simulink model "lineTwist"  (Simulink 8.5)
settings: Solver=ode15s  SolverMode=SingleTasking  StartTime=0.0  StopTime=0.1  MaxStep=0.0001  RelTol=1e-4  AbsTol=1e-6
libraries: powerlib x46
settings Model: Creator=Dr. Lotfifard  LastModifiedBy=PC
settings SolverCC: InitialStep=0.000001
settings DataIOCC: LimitDataPoints=off
settings OptimizationCC: BlockReduction=off  BooleanDataType=off
settings DebuggingCC: SaveWithParameterizedLinksMsg=none  SignalResolutionControl=TryResolveAllWithWarning  MultiTaskDSMMsg=warning  MultiTaskCondExecSysMsg=none  FcnCallInpInsideContextMsg=UseLocalSettings
settings HardwareCC: TargetUnknown=on

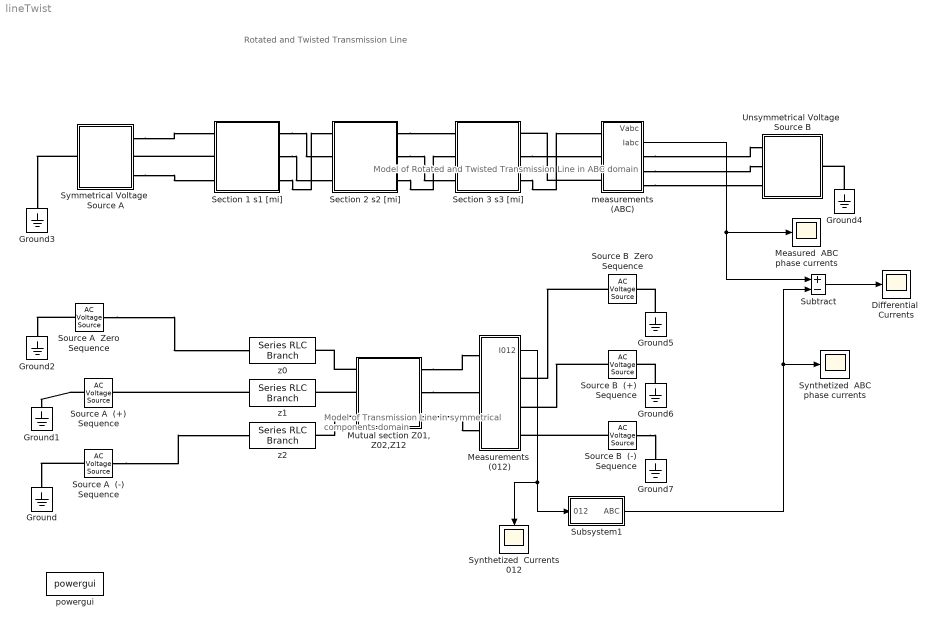
== system lineTwist ==
  note: Rotated and Twisted Transmission Line
  note: Model of Transmission Line
      |     in symmetrical components domain
  note: Model of Rotated and Twisted Transmission Line
      | in ABC domain
  Differential  Currents : Scope
      settings: TickLabels=on  TimeRange=0.07000000000000001  YMin=-10  YMax=10
  Ground{,1..7} (8 alike) : powerlib/Elements/Ground  LConnTagsString=a
  Measured  ABC phase currents : Scope
      settings: TickLabels=on  TimeRange=0.07000000000000001  YMin=-500  YMax=500  SaveName=ScopeData2
  Measurements  (012) : Subsystem
  "Mutual section Z01, Z02,Z12" : Subsystem
  Section 1 s1 [mi] : Subsystem
  Section 2 s2 [mi] : Subsystem
  Section 3 s3 [mi] : Subsystem
  Source A  (+) Sequence : powerlib/Electrical Sources/AC Voltage Source  Tag=PoWeRsYsTeMbLoCk  Amplitude=100  Phase=0  Frequency=60  SampleTime=0  Measurements=None
  Source A  (-) Sequence : powerlib/Electrical Sources/AC Voltage Source  Tag=PoWeRsYsTeMbLoCk  Amplitude=100  Phase=0  Frequency=60  SampleTime=0  Measurements=None
  Source A  Zero Sequence : powerlib/Electrical Sources/AC Voltage Source  Tag=PoWeRsYsTeMbLoCk  Amplitude=100  Phase=0  Frequency=60  SampleTime=0  Measurements=None
  Source B  (+) Sequence : powerlib/Electrical Sources/AC Voltage Source  Tag=PoWeRsYsTeMbLoCk  Amplitude=100  Phase=0  Frequency=60  SampleTime=0  Measurements=None
  Source B  (-) Sequence : powerlib/Electrical Sources/AC Voltage Source  Tag=PoWeRsYsTeMbLoCk  Amplitude=100  Phase=0  Frequency=60  SampleTime=0  Measurements=None
  Source B  Zero Sequence : powerlib/Electrical Sources/AC Voltage Source  Tag=PoWeRsYsTeMbLoCk  Amplitude=100  Phase=0  Frequency=60  SampleTime=0  Measurements=None
  Subsystem1 : Subsystem
  Subtract : Sum  Inputs=+-  SaturateOnIntegerOverflow=on  InputSameDT=on  OutDataTypeStr=Inherit: Same as first input
  Symmetrical Voltage  Source A : Subsystem
  Synthetized  ABC phase currents : Scope
      settings: TickLabels=on  TimeRange=0.07000000000000001  YMin=-500  YMax=500  SaveName=ScopeData3
  Synthetized  Currents 012 : Scope
      settings: TickLabels=on  TimeRange=0.07000000000000001
  Unsymmetrical Voltage  Source B : Subsystem
  measurements (ABC) : Subsystem
  powergui : powerlib/powergui  SimulationMode=Continuous  SolverType=Tustin/Backward Euler (TBE)  SampleTime=0  frequency=60  SPID=off  DisableSnubberDevices=off  DisableRonSwitches=off  DisableVfSwitches=off  SwTol=0  DisplayEquations=off  Interpol=off  methode=off  Ts=0  FunctionMessages=off  echomessages=off  HookPort=off  EnableUseOfTLC=off  x0status=blocks  frequencyindice=60  Pbase=100e6  ErrMax=1e-4  Iterations=50  UnitsV=kV  UnitsW=MW  buscounter=0  RestoreLinks=warning  ResistiveCurrentMeasurement=off  Frange=[0:2:500]  Ylog=off  Xlog=on  ShowGrid=off  save=off  variable=ZData  structure=0  ZoomFFT=on  StartTime=0.0  cycles=1  DisplayStyle=1  fundamental=60  FreqAxis=off  MaxFrequency=1000  frequencyindicesteady=1  RmsSteady=1  display=off
  z0 : powerlib/Elements/Series RLC Branch  LConnTagsString=__new0  RConnTagsString=__new0  BranchType=RLC  Resistance=1  Inductance=1e-3  SetiL0=off  InitialCurrent=0  Capacitance=1e-6  Setx0=off  InitialVoltage=0  Measurements=None
  z1 : powerlib/Elements/Series RLC Branch  LConnTagsString=__new0  RConnTagsString=__new0  BranchType=RLC  Resistance=1  Inductance=1e-3  SetiL0=off  InitialCurrent=0  Capacitance=1e-6  Setx0=off  InitialVoltage=0  Measurements=None
  z2 : powerlib/Elements/Series RLC Branch  LConnTagsString=__new0  RConnTagsString=__new0  BranchType=RLC  Resistance=1  Inductance=1e-3  SetiL0=off  InitialCurrent=0  Capacitance=1e-6  Setx0=off  InitialVoltage=0  Measurements=None
  wires:
  Subtract/1 -> Differential  Currents/1
  Subsystem1/1(ABC) -> Synthetized  ABC phase currents/1, Subtract/2
  Measurements  (012)/1(I012) -> Subsystem1/1(012), Synthetized  Currents 012/1
  measurements (ABC)/2(Iabc) -> Measured  ABC phase currents/1, Subtract/1
  connections:
  Source A  Zero Sequence/LConn1 -- Ground2/LConn1
  Source A  (+) Sequence/LConn1 -- Ground1/LConn1
  Source A  (-) Sequence/LConn1 -- Ground/LConn1
  Ground6/LConn1 -- Source B  (+) Sequence/LConn1
  Source B  (-) Sequence/LConn1 -- Ground7/LConn1
  Ground5/LConn1 -- Source B  Zero Sequence/LConn1
  "Mutual section Z01, Z02,Z12"/LConn1 -- z0/RConn1
  Source A  (-) Sequence/RConn1 -- z2/LConn1
  "Mutual section Z01, Z02,Z12"/LConn2 -- z1/RConn1
  "Mutual section Z01, Z02,Z12"/LConn3 -- z2/RConn1
  z1/LConn1 -- Source A  (+) Sequence/RConn1
  Source A  Zero Sequence/RConn1 -- z0/LConn1
  Symmetrical Voltage  Source A/RConn1 -- Section 1 s1 [mi]/LConn1
  Section 3 s3 [mi]/RConn3 -- measurements (ABC)/LConn1
  Section 1 s1 [mi]/LConn2 -- Symmetrical Voltage  Source A/RConn2
  Symmetrical Voltage  Source A/RConn3 -- Section 1 s1 [mi]/LConn3
  Symmetrical Voltage  Source A/LConn1 -- Ground3/LConn1
  Section 1 s1 [mi]/RConn1 -- Section 2 s2 [mi]/LConn2
  Section 1 s1 [mi]/RConn3 -- Section 2 s2 [mi]/LConn1
  Section 1 s1 [mi]/RConn2 -- Section 2 s2 [mi]/LConn3
  measurements (ABC)/RConn2 -- Unsymmetrical Voltage  Source B/RConn2
  measurements (ABC)/RConn3 -- Unsymmetrical Voltage  Source B/RConn3
  measurements (ABC)/RConn1 -- Unsymmetrical Voltage  Source B/RConn1
  "Mutual section Z01, Z02,Z12"/RConn1 -- Measurements  (012)/LConn1
  Ground4/LConn1 -- Unsymmetrical Voltage  Source B/LConn1
  Source B  Zero Sequence/RConn1 -- Measurements  (012)/RConn1
  "Mutual section Z01, Z02,Z12"/RConn2 -- Measurements  (012)/LConn2
  Source B  (-) Sequence/RConn1 -- Measurements  (012)/RConn3
  "Mutual section Z01, Z02,Z12"/RConn3 -- Measurements  (012)/LConn3
  Source B  (+) Sequence/RConn1 -- Measurements  (012)/RConn2
  Section 2 s2 [mi]/RConn1 -- Section 3 s3 [mi]/LConn1
  Section 2 s2 [mi]/RConn2 -- Section 3 s3 [mi]/LConn3
  Section 2 s2 [mi]/RConn3 -- Section 3 s3 [mi]/LConn2
  measurements (ABC)/LConn3 -- Section 3 s3 [mi]/RConn1
  Section 3 s3 [mi]/RConn2 -- measurements (ABC)/LConn2

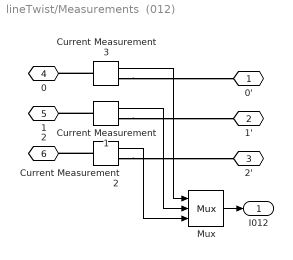
== system lineTwist/Measurements  (012) ==
  Current Measurement1 : powerlib/Measurements/Current Measurement  PhasorSimulation=off  OutputType=Complex  PSBequivalent=0
  Current Measurement2 : powerlib/Measurements/Current Measurement  PhasorSimulation=off  OutputType=Complex  PSBequivalent=0
  Current Measurement3 : powerlib/Measurements/Current Measurement  PhasorSimulation=off  OutputType=Complex  PSBequivalent=0
  Mux : Mux  Inputs=3
  0' : PMIOPort  Port=1  Side=Right
  1' : PMIOPort  Port=2  Side=Right
  2' : PMIOPort  Port=3  Side=Right
  0 : PMIOPort  Port=4  Side=Left
  1 : PMIOPort  Port=5  Side=Left
  2 : PMIOPort  Port=6  Side=Left
  I012 : Outport  InitialOutput=0
  wires:
  Current Measurement3/1 -> Mux/1
  Current Measurement1/1 -> Mux/2
  Mux/1 -> I012/1
  Current Measurement2/1 -> Mux/3
  connections:
  Current Measurement3/RConn1 -- 0'/RConn1
  Current Measurement1/RConn1 -- 1'/RConn1
  Current Measurement2/RConn1 -- 2'/RConn1
  Current Measurement2/LConn1 -- 2/RConn1
  Current Measurement1/LConn1 -- 1/RConn1
  Current Measurement3/LConn1 -- 0/RConn1

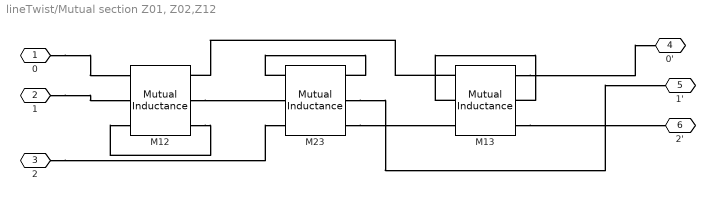
== system lineTwist/Mutual section Z01, Z02,Z12 ==
  M12 : powerlib/Elements/Mutual Inductance  LConnTagsString=a|b|c  RConnTagsString=A|B|C  TypeOfMutual=Two or three windings with equal mutual terms  NumberOfWindings=3  SelfImpedance1=[1.1 1.1e-03]  SelfImpedance2=[ 1.1 1.1e-03]  ThreeWindings=on  SelfImpedance3=[ 1.1 1.1e-03]  MutualImpedance=[1.0 1.0e-03]  InductanceMatrix="[1.0 0.9  0.9 ;  0.9 1.0  0.9;  0.9 0.9 1.0 ] * 1e-3"  ResistanceMatrix="[1.0 0.9  0.9 ;  0.9 1.0  0.9;  0.9 0.9 1.0 ]"  Measurements=None
      settings: AttributesFormatString=\n
  M13 : powerlib/Elements/Mutual Inductance  LConnTagsString=a|b|c  RConnTagsString=A|B|C  TypeOfMutual=Two or three windings with equal mutual terms  NumberOfWindings=3  SelfImpedance1=[1.1 1.1e-03]  SelfImpedance2=[ 1.1 1.1e-03]  ThreeWindings=on  SelfImpedance3=[ 1.1 1.1e-03]  MutualImpedance=[1.0 1.0e-03]  InductanceMatrix="[1.0 0.9  0.9 ;  0.9 1.0  0.9;  0.9 0.9 1.0 ] * 1e-3"  ResistanceMatrix="[1.0 0.9  0.9 ;  0.9 1.0  0.9;  0.9 0.9 1.0 ]"  Measurements=None
      settings: AttributesFormatString=\n
  M23 : powerlib/Elements/Mutual Inductance  LConnTagsString=a|b|c  RConnTagsString=A|B|C  TypeOfMutual=Two or three windings with equal mutual terms  NumberOfWindings=3  SelfImpedance1=[1.1 1.1e-03]  SelfImpedance2=[ 1.1 1.1e-03]  ThreeWindings=on  SelfImpedance3=[ 1.1 1.1e-03]  MutualImpedance=[1.0 1.0e-03]  InductanceMatrix="[1.0 0.9  0.9 ;  0.9 1.0  0.9;  0.9 0.9 1.0 ] * 1e-3"  ResistanceMatrix="[1.0 0.9  0.9 ;  0.9 1.0  0.9;  0.9 0.9 1.0 ]"  Measurements=None
      settings: AttributesFormatString=\n
  0 : PMIOPort  Port=1  Side=Left
  1 : PMIOPort  Port=2  Side=Left
  2 : PMIOPort  Port=3  Side=Left
  0' : PMIOPort  Port=4  Side=Right
  1' : PMIOPort  Port=5  Side=Right
  2' : PMIOPort  Port=6  Side=Right
  connections:
  0/RConn1 -- M12/LConn1
  1/RConn1 -- M12/LConn2
  2/RConn1 -- M23/LConn3
  M12/RConn3 -- M12/LConn3
  M23/LConn1 -- M23/RConn1
  M13/LConn2 -- M13/RConn2
  M12/RConn2 -- M23/LConn2
  M13/LConn1 -- M12/RConn1
  M23/RConn3 -- M13/LConn3
  M23/RConn2 -- 1'/RConn1
  M13/RConn1 -- 0'/RConn1
  M13/RConn3 -- 2'/RConn1

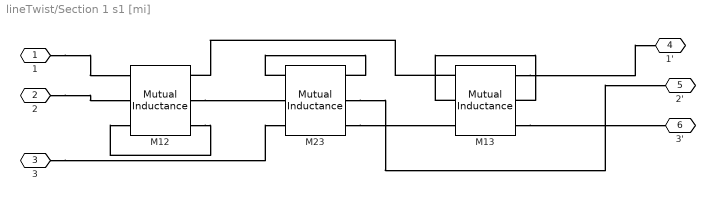
== system lineTwist/Section 1 s1 [mi] ==
  M12 : powerlib/Elements/Mutual Inductance  LConnTagsString=a|b|c  RConnTagsString=A|B|C  TypeOfMutual=Two or three windings with equal mutual terms  NumberOfWindings=3  SelfImpedance1=[1.1 1.1e-03]  SelfImpedance2=[ 1.1 1.1e-03]  ThreeWindings=on  SelfImpedance3=[ 1.1 1.1e-03]  MutualImpedance=[1.0 1.0e-03]  InductanceMatrix="[1.0 0.9  0.9 ;  0.9 1.0  0.9;  0.9 0.9 1.0 ] * 1e-3"  ResistanceMatrix="[1.0 0.9  0.9 ;  0.9 1.0  0.9;  0.9 0.9 1.0 ]"  Measurements=None
      settings: AttributesFormatString=\n
  M13 : powerlib/Elements/Mutual Inductance  LConnTagsString=a|b|c  RConnTagsString=A|B|C  TypeOfMutual=Two or three windings with equal mutual terms  NumberOfWindings=3  SelfImpedance1=[1.1 1.1e-03]  SelfImpedance2=[ 1.1 1.1e-03]  ThreeWindings=on  SelfImpedance3=[ 1.1 1.1e-03]  MutualImpedance=[1.0 1.0e-03]  InductanceMatrix="[1.0 0.9  0.9 ;  0.9 1.0  0.9;  0.9 0.9 1.0 ] * 1e-3"  ResistanceMatrix="[1.0 0.9  0.9 ;  0.9 1.0  0.9;  0.9 0.9 1.0 ]"  Measurements=None
      settings: AttributesFormatString=\n
  M23 : powerlib/Elements/Mutual Inductance  LConnTagsString=a|b|c  RConnTagsString=A|B|C  TypeOfMutual=Two or three windings with equal mutual terms  NumberOfWindings=3  SelfImpedance1=[1.1 1.1e-03]  SelfImpedance2=[ 1.1 1.1e-03]  ThreeWindings=on  SelfImpedance3=[ 1.1 1.1e-03]  MutualImpedance=[1.0 1.0e-03]  InductanceMatrix="[1.0 0.9  0.9 ;  0.9 1.0  0.9;  0.9 0.9 1.0 ] * 1e-3"  ResistanceMatrix="[1.0 0.9  0.9 ;  0.9 1.0  0.9;  0.9 0.9 1.0 ]"  Measurements=None
      settings: AttributesFormatString=\n
  1 : PMIOPort  Port=1  Side=Left
  2 : PMIOPort  Port=2  Side=Left
  3 : PMIOPort  Port=3  Side=Left
  1' : PMIOPort  Port=4  Side=Right
  2' : PMIOPort  Port=5  Side=Right
  3' : PMIOPort  Port=6  Side=Right
  connections:
  1/RConn1 -- M12/LConn1
  2/RConn1 -- M12/LConn2
  3/RConn1 -- M23/LConn3
  M12/RConn3 -- M12/LConn3
  M23/LConn1 -- M23/RConn1
  M13/LConn2 -- M13/RConn2
  M12/RConn2 -- M23/LConn2
  M13/LConn1 -- M12/RConn1
  M23/RConn3 -- M13/LConn3
  M23/RConn2 -- 2'/RConn1
  M13/RConn1 -- 1'/RConn1
  M13/RConn3 -- 3'/RConn1

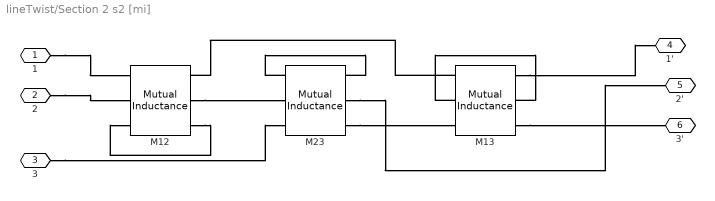
== system lineTwist/Section 2 s2 [mi] ==
  M12 : powerlib/Elements/Mutual Inductance  LConnTagsString=a|b|c  RConnTagsString=A|B|C  TypeOfMutual=Two or three windings with equal mutual terms  NumberOfWindings=3  SelfImpedance1=[1.1 1.1e-03]  SelfImpedance2=[ 1.1 1.1e-03]  ThreeWindings=on  SelfImpedance3=[ 1.1 1.1e-03]  MutualImpedance=[1.0 1.0e-03]  InductanceMatrix="[1.0 0.9  0.9 ;  0.9 1.0  0.9;  0.9 0.9 1.0 ] * 1e-3"  ResistanceMatrix="[1.0 0.9  0.9 ;  0.9 1.0  0.9;  0.9 0.9 1.0 ]"  Measurements=None
      settings: AttributesFormatString=\n
  M13 : powerlib/Elements/Mutual Inductance  LConnTagsString=a|b|c  RConnTagsString=A|B|C  TypeOfMutual=Two or three windings with equal mutual terms  NumberOfWindings=3  SelfImpedance1=[1.1 1.1e-03]  SelfImpedance2=[ 1.1 1.1e-03]  ThreeWindings=on  SelfImpedance3=[ 1.1 1.1e-03]  MutualImpedance=[1.0 1.0e-03]  InductanceMatrix="[1.0 0.9  0.9 ;  0.9 1.0  0.9;  0.9 0.9 1.0 ] * 1e-3"  ResistanceMatrix="[1.0 0.9  0.9 ;  0.9 1.0  0.9;  0.9 0.9 1.0 ]"  Measurements=None
      settings: AttributesFormatString=\n
  M23 : powerlib/Elements/Mutual Inductance  LConnTagsString=a|b|c  RConnTagsString=A|B|C  TypeOfMutual=Two or three windings with equal mutual terms  NumberOfWindings=3  SelfImpedance1=[1.1 1.1e-03]  SelfImpedance2=[ 1.1 1.1e-03]  ThreeWindings=on  SelfImpedance3=[ 1.1 1.1e-03]  MutualImpedance=[1.0 1.0e-03]  InductanceMatrix="[1.0 0.9  0.9 ;  0.9 1.0  0.9;  0.9 0.9 1.0 ] * 1e-3"  ResistanceMatrix="[1.0 0.9  0.9 ;  0.9 1.0  0.9;  0.9 0.9 1.0 ]"  Measurements=None
      settings: AttributesFormatString=\n
  1 : PMIOPort  Port=1  Side=Left
  2 : PMIOPort  Port=2  Side=Left
  3 : PMIOPort  Port=3  Side=Left
  1' : PMIOPort  Port=4  Side=Right
  2' : PMIOPort  Port=5  Side=Right
  3' : PMIOPort  Port=6  Side=Right
  connections:
  1/RConn1 -- M12/LConn1
  M12/RConn2 -- M23/LConn2
  M13/LConn2 -- M13/RConn2
  M23/LConn1 -- M23/RConn1
  3/RConn1 -- M23/LConn3
  M12/RConn3 -- M12/LConn3
  M13/RConn1 -- 1'/RConn1
  2/RConn1 -- M12/LConn2
  M13/LConn1 -- M12/RConn1
  M23/RConn3 -- M13/LConn3
  M23/RConn2 -- 2'/RConn1
  M13/RConn3 -- 3'/RConn1

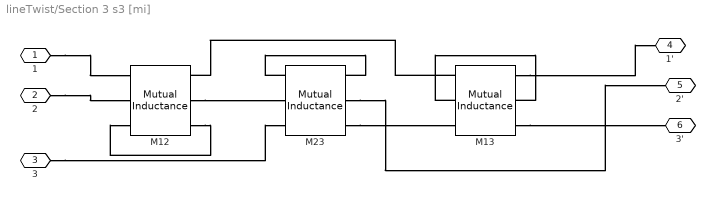
== system lineTwist/Section 3 s3 [mi] ==
  M12 : powerlib/Elements/Mutual Inductance  LConnTagsString=a|b|c  RConnTagsString=A|B|C  TypeOfMutual=Two or three windings with equal mutual terms  NumberOfWindings=3  SelfImpedance1=[1.1 1.1e-03]  SelfImpedance2=[ 1.1 1.1e-03]  ThreeWindings=on  SelfImpedance3=[ 1.1 1.1e-03]  MutualImpedance=[1.0 1.0e-03]  InductanceMatrix="[1.0 0.9  0.9 ;  0.9 1.0  0.9;  0.9 0.9 1.0 ] * 1e-3"  ResistanceMatrix="[1.0 0.9  0.9 ;  0.9 1.0  0.9;  0.9 0.9 1.0 ]"  Measurements=None
      settings: AttributesFormatString=\n
  M13 : powerlib/Elements/Mutual Inductance  LConnTagsString=a|b|c  RConnTagsString=A|B|C  TypeOfMutual=Two or three windings with equal mutual terms  NumberOfWindings=3  SelfImpedance1=[1.1 1.1e-03]  SelfImpedance2=[ 1.1 1.1e-03]  ThreeWindings=on  SelfImpedance3=[ 1.1 1.1e-03]  MutualImpedance=[1.0 1.0e-03]  InductanceMatrix="[1.0 0.9  0.9 ;  0.9 1.0  0.9;  0.9 0.9 1.0 ] * 1e-3"  ResistanceMatrix="[1.0 0.9  0.9 ;  0.9 1.0  0.9;  0.9 0.9 1.0 ]"  Measurements=None
      settings: AttributesFormatString=\n
  M23 : powerlib/Elements/Mutual Inductance  LConnTagsString=a|b|c  RConnTagsString=A|B|C  TypeOfMutual=Two or three windings with equal mutual terms  NumberOfWindings=3  SelfImpedance1=[1.1 1.1e-03]  SelfImpedance2=[ 1.1 1.1e-03]  ThreeWindings=on  SelfImpedance3=[ 1.1 1.1e-03]  MutualImpedance=[1.0 1.0e-03]  InductanceMatrix="[1.0 0.9  0.9 ;  0.9 1.0  0.9;  0.9 0.9 1.0 ] * 1e-3"  ResistanceMatrix="[1.0 0.9  0.9 ;  0.9 1.0  0.9;  0.9 0.9 1.0 ]"  Measurements=None
      settings: AttributesFormatString=\n
  1 : PMIOPort  Port=1  Side=Left
  2 : PMIOPort  Port=2  Side=Left
  3 : PMIOPort  Port=3  Side=Left
  1' : PMIOPort  Port=4  Side=Right
  2' : PMIOPort  Port=5  Side=Right
  3' : PMIOPort  Port=6  Side=Right
  connections:
  1/RConn1 -- M12/LConn1
  M12/RConn2 -- M23/LConn2
  M13/LConn2 -- M13/RConn2
  M23/LConn1 -- M23/RConn1
  3/RConn1 -- M23/LConn3
  M12/RConn3 -- M12/LConn3
  M13/RConn1 -- 1'/RConn1
  2/RConn1 -- M12/LConn2
  M13/LConn1 -- M12/RConn1
  M23/RConn3 -- M13/LConn3
  M23/RConn2 -- 2'/RConn1
  M13/RConn3 -- 3'/RConn1

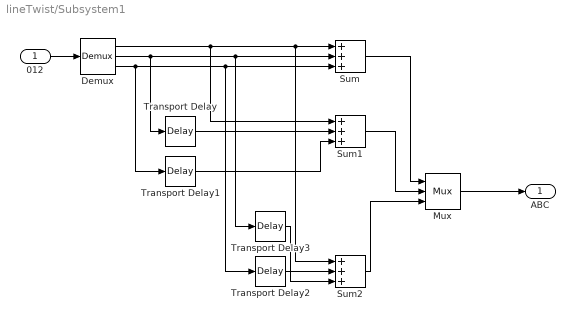
== system lineTwist/Subsystem1 ==
  012 : Inport
  Demux : Demux  Outputs=3
  Mux : Mux  Inputs=3
  Sum : Sum  Inputs=+++  SaturateOnIntegerOverflow=on  InputSameDT=on  OutDataTypeStr=Inherit: Same as first input
  Sum1 : Sum  Inputs=+++  SaturateOnIntegerOverflow=on  InputSameDT=on  OutDataTypeStr=Inherit: Same as first input
  Sum2 : Sum  Inputs=+++  SaturateOnIntegerOverflow=on  InputSameDT=on  OutDataTypeStr=Inherit: Same as first input
  Transport Delay : TransportDelay  DelayTime=1/(3*60)
  Transport Delay1 : TransportDelay  DelayTime=2/(3*60)
  Transport Delay2 : TransportDelay  DelayTime=1/(3*60)
  Transport Delay3 : TransportDelay  DelayTime=2/(3*60)
  ABC : Outport  InitialOutput=0
  wires:
  012/1 -> Demux/1
  Demux/2 -> Transport Delay/1, Sum/2, Transport Delay3/1
  Demux/3 -> Transport Delay1/1, Sum/3, Transport Delay2/1
  Demux/1 -> Sum1/1, Sum/1, Sum2/1
  Transport Delay/1 -> Sum1/2
  Transport Delay1/1 -> Sum1/3
  Transport Delay2/1 -> Sum2/3
  Transport Delay3/1 -> Sum2/2
  Mux/1 -> ABC/1
  Sum2/1 -> Mux/3
  Sum1/1 -> Mux/2
  Sum/1 -> Mux/1

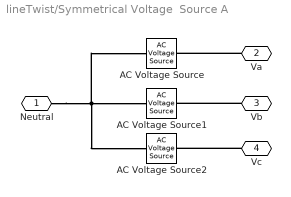
== system lineTwist/Symmetrical Voltage  Source A ==
  AC Voltage Source : powerlib/Electrical Sources/AC Voltage Source  Tag=PoWeRsYsTeMbLoCk  Amplitude=100  Phase=0  Frequency=60  SampleTime=0  Measurements=None
  AC Voltage Source1 : powerlib/Electrical Sources/AC Voltage Source  Tag=PoWeRsYsTeMbLoCk  Amplitude=100  Phase=0  Frequency=60  SampleTime=0  Measurements=None
  AC Voltage Source2 : powerlib/Electrical Sources/AC Voltage Source  Tag=PoWeRsYsTeMbLoCk  Amplitude=100  Phase=0  Frequency=60  SampleTime=0  Measurements=None
  Neutral : PMIOPort  Port=1  Side=Left
  Va : PMIOPort  Port=2  Side=Right
  Vb : PMIOPort  Port=3  Side=Right
  Vc : PMIOPort  Port=4  Side=Right
  connections:
  Neutral/RConn1 -- AC Voltage Source1/LConn1 -- AC Voltage Source/LConn1 -- AC Voltage Source2/LConn1
  Vb/RConn1 -- AC Voltage Source1/RConn1
  Va/RConn1 -- AC Voltage Source/RConn1
  Vc/RConn1 -- AC Voltage Source2/RConn1

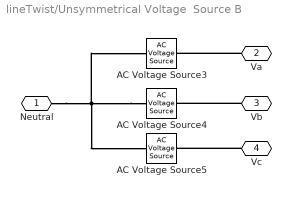
== system lineTwist/Unsymmetrical Voltage  Source B ==
  AC Voltage Source3 : powerlib/Electrical Sources/AC Voltage Source  Tag=PoWeRsYsTeMbLoCk  Amplitude=100  Phase=0  Frequency=60  SampleTime=0  Measurements=None
  AC Voltage Source4 : powerlib/Electrical Sources/AC Voltage Source  Tag=PoWeRsYsTeMbLoCk  Amplitude=100  Phase=0  Frequency=60  SampleTime=0  Measurements=None
  AC Voltage Source5 : powerlib/Electrical Sources/AC Voltage Source  Tag=PoWeRsYsTeMbLoCk  Amplitude=100  Phase=0  Frequency=60  SampleTime=0  Measurements=None
  Neutral : PMIOPort  Port=1  Side=Left
  Va : PMIOPort  Port=2  Side=Right
  Vb : PMIOPort  Port=3  Side=Right
  Vc : PMIOPort  Port=4  Side=Right
  connections:
  AC Voltage Source4/LConn1 -- AC Voltage Source3/LConn1 -- AC Voltage Source5/LConn1 -- Neutral/RConn1
  Vb/RConn1 -- AC Voltage Source4/RConn1
  Vc/RConn1 -- AC Voltage Source5/RConn1
  Va/RConn1 -- AC Voltage Source3/RConn1

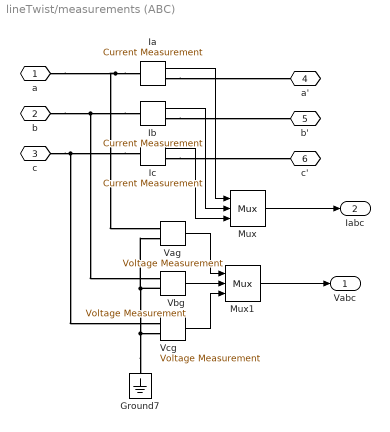
== system lineTwist/measurements (ABC) ==
  Ground7 : powerlib/Elements/Ground  LConnTagsString=a
  Ia : powerlib/Measurements/Current Measurement  PhasorSimulation=off  OutputType=Complex  PSBequivalent=0
  Ib : powerlib/Measurements/Current Measurement  PhasorSimulation=off  OutputType=Complex  PSBequivalent=0
  Ic : powerlib/Measurements/Current Measurement  PhasorSimulation=off  OutputType=Complex  PSBequivalent=0
  Mux : Mux  Inputs=3
  Mux1 : Mux  Inputs=3
  Vag : powerlib/Measurements/Voltage Measurement  PhasorSimulation=off  OutputType=Complex  PSBequivalent=0
  Vbg : powerlib/Measurements/Voltage Measurement  PhasorSimulation=off  OutputType=Complex  PSBequivalent=0
  Vcg : powerlib/Measurements/Voltage Measurement  PhasorSimulation=off  OutputType=Complex  PSBequivalent=0
  a : PMIOPort  Port=1  Side=Left
  b : PMIOPort  Port=2  Side=Left
  c : PMIOPort  Port=3  Side=Left
  a' : PMIOPort  Port=4  Side=Right
  b' : PMIOPort  Port=5  Side=Right
  c' : PMIOPort  Port=6  Side=Right
  Vabc : Outport  InitialOutput=0
  Iabc : Outport  Port=2  InitialOutput=0
  wires:
  Vcg/1 -> Mux1/3
  Vag/1 -> Mux1/1
  Vbg/1 -> Mux1/2
  Mux1/1 -> Vabc/1
  Mux/1 -> Iabc/1
  Ia/1 -> Mux/1
  Ib/1 -> Mux/2
  Ic/1 -> Mux/3
  connections:
  Ia/LConn1 -- Vag/LConn1 -- a/RConn1
  Ib/LConn1 -- Vbg/LConn1 -- b/RConn1
  Ic/LConn1 -- Vcg/LConn1 -- c/RConn1
  Ia/RConn1 -- a'/RConn1
  Ib/RConn1 -- b'/RConn1
  Ic/RConn1 -- c'/RConn1
  Ground7/LConn1 -- Vcg/LConn2 -- Vag/LConn2 -- Vbg/LConn2
